simulink model "ban5"  (R2018b)
settings: Solver=FixedStepAuto  StartTime=0.0  StopTime=10  FixedStep=0.001  RelTol=1e-3
libraries: simulink x1
settings Model: Creator=User  LastModifiedBy=User

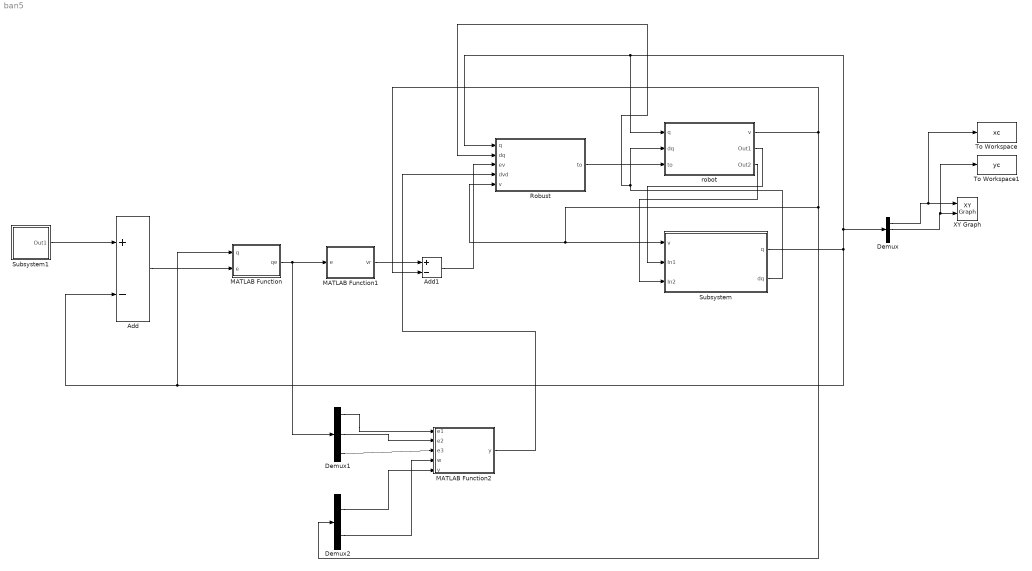
== system ban5 ==
  Add : Sum  Inputs=+-
  Add1 : Sum  Inputs=+-
  Demux : Demux  Outputs=3
  Demux1 : Demux  Outputs=3
  Demux2 : Demux  Outputs=2
  MATLAB Function : MATLAB Function  TreatAsAtomicUnit=on
  MATLAB Function1 : MATLAB Function  TreatAsAtomicUnit=on
  MATLAB Function2 : MATLAB Function  TreatAsAtomicUnit=on
  Robust : Subsystem
  Subsystem : Subsystem
  Subsystem1 : Subsystem
  To Workspace : ToWorkspace  VariableName=xc  SampleTime=-1
  To Workspace1 : ToWorkspace  VariableName=yc  SampleTime=-1
  XY Graph : simulink/Sinks/XY Graph  xmin=-4  xmax=4  ymin=-4  ymax=4  st=0.005
  robot : Subsystem
  wires:
  Subsystem1/1(Out1) -> Add/1
  Subsystem/1(q) -> robot/1(q), Robust/1(q), Demux/1, MATLAB Function/1(q), Add/2
  Add/1 -> MATLAB Function/2(e)
  MATLAB Function/1(qe) -> Demux1/1, MATLAB Function1/1(e)
  robot/1(v) -> Demux2/1, Subsystem/1(v), Robust/5(v), Add1/2
  Add1/1 -> Robust/3(ev)
  Subsystem/2(dq) -> robot/2(dq), Robust/2(dq)
  Demux/1 -> To Workspace/1, XY Graph/1
  Demux/2 -> To Workspace1/1, XY Graph/2
  robot/2(Out1) -> Subsystem/2(In1)
  robot/3(Out2) -> Subsystem/3(In2)
  Demux1/1 -> MATLAB Function2/1(e1)
  Demux1/2 -> MATLAB Function2/2(e2)
  Demux1/3 -> MATLAB Function2/3(e3)
  Demux2/1 -> MATLAB Function2/5(v)
  Demux2/2 -> MATLAB Function2/4(w)
  Robust/1(to) -> robot/3(to)
  MATLAB Function2/1(y) -> Robust/4(dvd)
  MATLAB Function1/1(vr) -> Add1/1

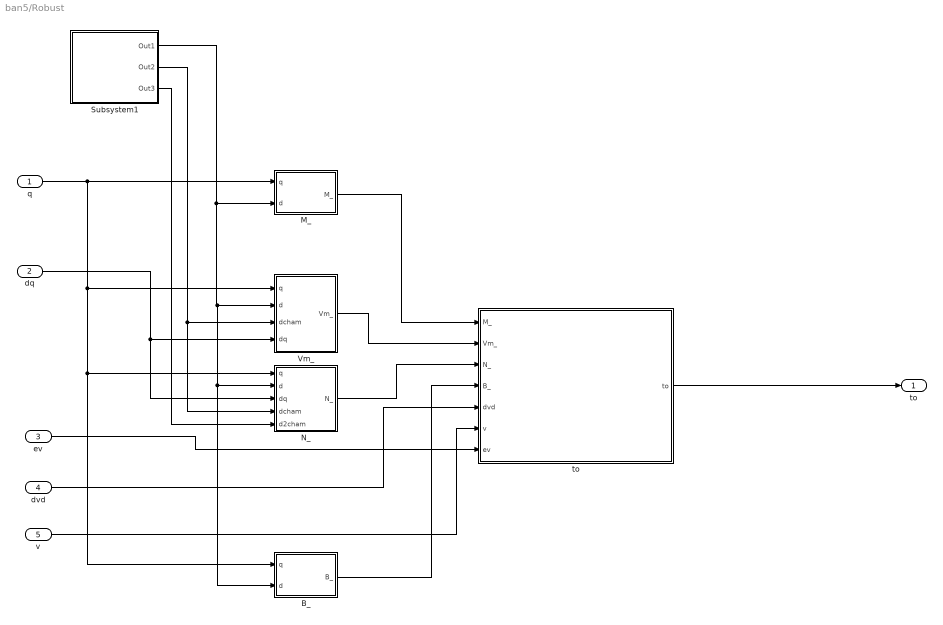
== system ban5/Robust ==
  q : Inport
  dq : Inport  Port=2
  ev : Inport  Port=3
  dvd : Inport  Port=4
  v : Inport  Port=5
  B_ : MATLAB Function  TreatAsAtomicUnit=on
  M_ : MATLAB Function  TreatAsAtomicUnit=on
  N_ : MATLAB Function  TreatAsAtomicUnit=on
  Subsystem1 : Subsystem
  Vm_ : MATLAB Function  TreatAsAtomicUnit=on
  "to " : MATLAB Function  TreatAsAtomicUnit=on
  to : Outport
  wires:
  dq/1 -> Vm_/4(dq), N_/3(dq)
  q/1 -> M_/1(q), Vm_/1(q), N_/1(q), B_/1(q)
  B_/1(B_) -> "to "/4(B_)
  N_/1(N_) -> "to "/3(N_)
  Vm_/1(Vm_) -> "to "/2(Vm_)
  M_/1(M_) -> "to "/1(M_)
  dvd/1 -> "to "/5(dvd)
  v/1 -> "to "/6(v)
  ev/1 -> "to "/7(ev)
  "to "/1(to) -> to/1
  Subsystem1/1(Out1) -> B_/2(d), N_/2(d), Vm_/2(d), M_/2(d)
  Subsystem1/2(Out2) -> N_/4(dcham), Vm_/3(dcham)
  Subsystem1/3(Out3) -> N_/5(d2cham)

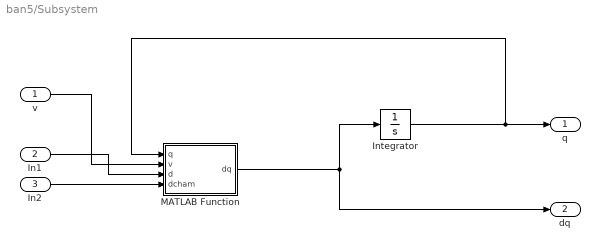
== system ban5/Subsystem ==
  v : Inport
  In1 : Inport  Port=2
  In2 : Inport  Port=3
  Integrator : Integrator  InitialCondition=[1.8852;-0.2772;3*pi/8]
  MATLAB Function : MATLAB Function  TreatAsAtomicUnit=on
  q : Outport
  dq : Outport  Port=2
  wires:
  Integrator/1 -> MATLAB Function/1(q), q/1
  MATLAB Function/1(dq) -> Integrator/1, dq/1
  v/1 -> MATLAB Function/2(v)
  In1/1 -> MATLAB Function/3(d)
  In2/1 -> MATLAB Function/4(dcham)

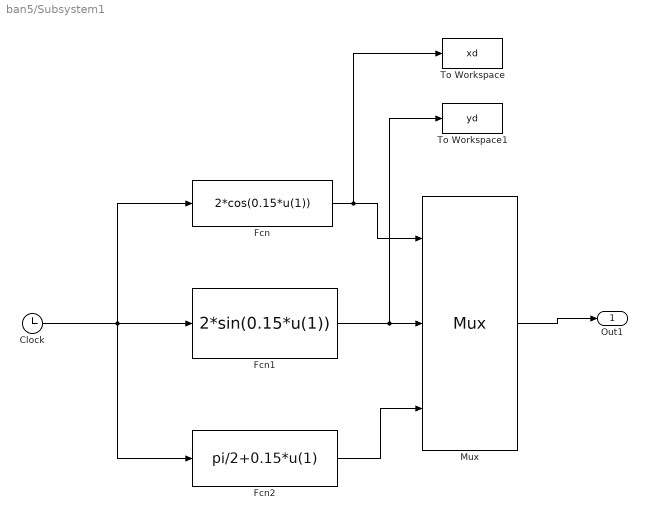
== system ban5/Subsystem1 ==
  Clock : Clock
  Fcn : Fcn  Expr=2*cos(0.15*u(1))
  Fcn1 : Fcn  Expr=2*sin(0.15*u(1))
  Fcn2 : Fcn  Expr=pi/2+0.15*u(1)
  Mux : Mux  Inputs=3
  To Workspace : ToWorkspace  VariableName=xd  SampleTime=-1
  To Workspace1 : ToWorkspace  VariableName=yd  SampleTime=-1
  Out1 : Outport
  wires:
  Clock/1 -> Fcn2/1, Fcn1/1, Fcn/1
  Fcn/1 -> To Workspace/1, Mux/1
  Fcn1/1 -> To Workspace1/1, Mux/2
  Fcn2/1 -> Mux/3
  Mux/1 -> Out1/1

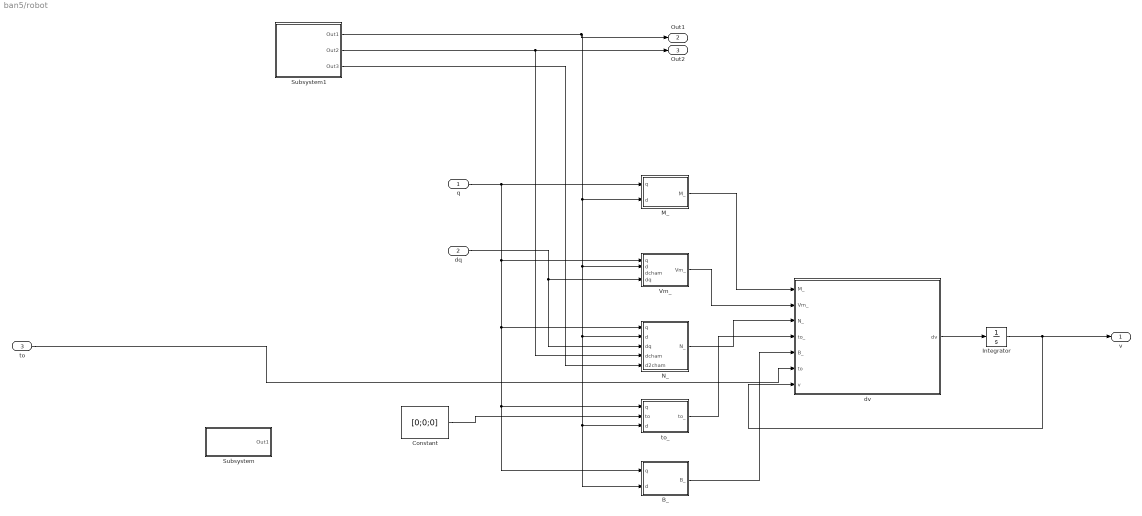
== system ban5/robot ==
  q : Inport
  dq : Inport  Port=2
  to : Inport  Port=3
  B_ : MATLAB Function  TreatAsAtomicUnit=on
  Constant : Constant  Value=[0;0;0]
  Integrator : Integrator  InitialCondition=[0;0]
  M_ : MATLAB Function  TreatAsAtomicUnit=on
  N_ : MATLAB Function  TreatAsAtomicUnit=on
  Subsystem : Subsystem
  Subsystem1 : Subsystem
  Vm_ : MATLAB Function  TreatAsAtomicUnit=on
  dv : MATLAB Function  TreatAsAtomicUnit=on
  to_ : MATLAB Function  TreatAsAtomicUnit=on
  v : Outport
  Out1 : Outport  Port=2
  Out2 : Outport  Port=3
  wires:
  M_/1(M_) -> dv/1(M_)
  Vm_/1(Vm_) -> dv/2(Vm_)
  N_/1(N_) -> dv/3(N_)
  to_/1(to_) -> dv/4(to_)
  B_/1(B_) -> dv/5(B_)
  dv/1(dv) -> Integrator/1
  Integrator/1 -> v/1, dv/7(v)
  q/1 -> B_/1(q), to_/1(q), N_/1(q), Vm_/1(q), M_/1(q)
  dq/1 -> N_/3(dq), Vm_/4(dq)
  to/1 -> dv/6(to)
  Subsystem1/1(Out1) -> Out1/1, B_/2(d), to_/3(d), N_/2(d), Vm_/2(d), M_/2(d)
  Subsystem1/3(Out3) -> N_/5(d2cham)
  Subsystem1/2(Out2) -> Out2/1, N_/4(dcham)
  Constant/1 -> to_/2(to)

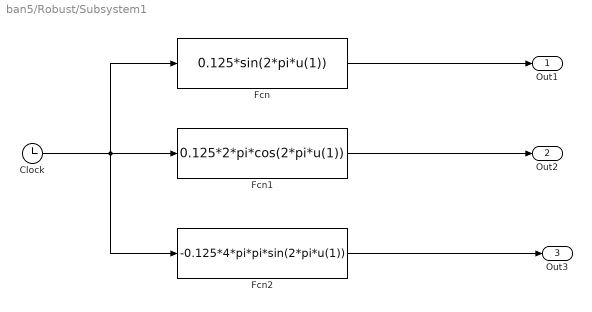
== system ban5/Robust/Subsystem1 ==
  Clock : Clock
  Fcn : Fcn  Expr=0.125*sin(2*pi*u(1))
  Fcn1 : Fcn  Expr=0.125*2*pi*cos(2*pi*u(1))
  Fcn2 : Fcn  Expr=-0.125*4*pi*pi*sin(2*pi*u(1))
  Out1 : Outport
  Out2 : Outport  Port=2
  Out3 : Outport  Port=3
  wires:
  Fcn2/1 -> Out3/1
  Fcn1/1 -> Out2/1
  Fcn/1 -> Out1/1
  Clock/1 -> Fcn2/1, Fcn1/1, Fcn/1

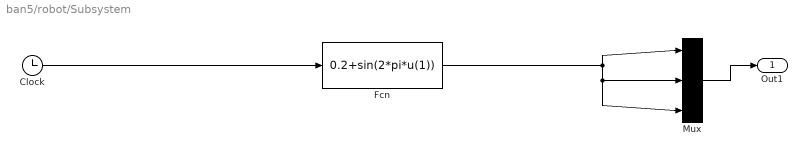
== system ban5/robot/Subsystem ==
  Clock : Clock
  Fcn : Fcn  Expr=0.2+sin(2*pi*u(1))
  Mux : Mux  Inputs=3
  Out1 : Outport
  wires:
  Clock/1 -> Fcn/1
  Fcn/1 -> Mux/3, Mux/2, Mux/1
  Mux/1 -> Out1/1

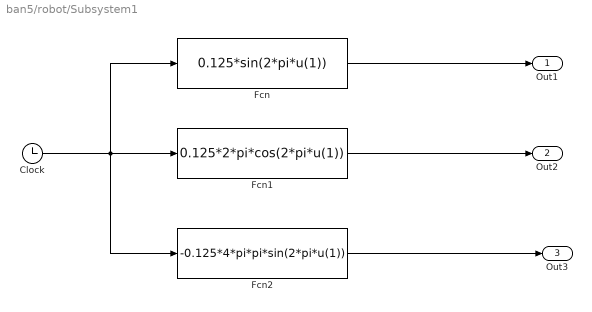
== system ban5/robot/Subsystem1 ==
  Clock : Clock
  Fcn : Fcn  Expr=0.125*sin(2*pi*u(1))
  Fcn1 : Fcn  Expr=0.125*2*pi*cos(2*pi*u(1))
  Fcn2 : Fcn  Expr=-0.125*4*pi*pi*sin(2*pi*u(1))
  Out1 : Outport
  Out2 : Outport  Port=2
  Out3 : Outport  Port=3
  wires:
  Fcn2/1 -> Out3/1
  Fcn1/1 -> Out2/1
  Fcn/1 -> Out1/1
  Clock/1 -> Fcn2/1, Fcn1/1, Fcn/1

== matlab function ban5/MATLAB Function ==
  data: q input; qe output; e input
function qe = fcn(q,e)
phi=q(3);
qe=[cos(phi) sin(phi) 0;-sin(phi) cos(phi) 0;0 0 1]*e;
end

== matlab function ban5/Subsystem/MATLAB Function ==
  data: q input; dq output; v input; d input; dcham input
function dq = fcn(q,v,d,dcham)
phi=[0 0 1]*q;
S=[cos(phi) -d*sin(phi);sin(phi) d*cos(phi);0 1];
n=[dcham*cos(phi);dcham*sin(phi);0];
dq=S*v+n;
end

== matlab function ban5/MATLAB Function1 ==
  data: e input; vr output
function vr=fcn(e)
vr=[0.3*cos([0 0 1]*e)+10*[1 0 0]*e;
    0.15+10*0.3*[0 1 0]*e+10*0.3*sin([0 0 1]*e)];
end

== matlab function ban5/robot/M_ ==
  data: q input; M_ output; d input
function M_ = fcn(q,d)
m=8;
I=0.7075+5*d^2;
M=[m 0 m*d*sin(q(3));
    0 m -m*d*cos(q(3));
    m*d*sin(q(3)) -m*d*cos(q(3)) I];
S=[cos(q(3)) -d*sin(q(3));
    sin(q(3)) d*cos(q(3));
    0 1];
M_=S'*M*S;
end

== matlab function ban5/robot/Vm_ ==
  data: q input; Vm_ output; d input; dcham input; dq input
function Vm_ = fcn(q,d,dcham,dq)
m=8;
I=0.7075+5*d^2;
M=[m 0 m*d*sin(q(3));
    0 m -m*d*cos(q(3));
    m*d*sin(q(3)) -m*d*cos(q(3)) I];
S=[cos(q(3)) -d*sin(q(3));
    sin(q(3)) d*cos(q(3));
    0 1];
dS=[-sin(q(3))*dq(3) -dcham*sin(q(3))-d*cos(q(3))*dq(3);
    cos(q(3))*dq(3) dcham*cos(q(3))-d*sin(q(3))*dq(3);
    0 0];
Vm=[0 0 m*d*dq(3)*cos(q(3));
    0 0 m*d*dq(3)*sin(q(3));
    0 0 0];
Vm_=S'*(M*dS+Vm*S);
end

== matlab function ban5/robot/N_ ==
  data: q input; N_ output; d input; dq input; dcham input; d2cham input
function N_ = fcn(q,d,dq,dcham,d2cham)
m=8;
I=0.7075+5*d^2;
M=[m 0 m*d*sin(q(3));
    0 m -m*d*cos(q(3));
    m*d*sin(q(3)) -m*d*cos(q(3)) I];
S=[cos(q(3)) -d*sin(q(3));
    sin(q(3)) d*cos(q(3));
    0 1];
Vm=[0 0 m*d*dq(3)*cos(q(3));
    0 0 m*d*dq(3)*sin(q(3));
    0 0 0];
n=[dcham*cos(q(3));dcham*sin(q(3));0];
dn=[d2cham*cos(q(3))+dcham*dq(3)*-sin(q(3));
    d2cham*sin(q(3))+dcham*dq(3)*cos(q(3));
    0];
N_=S'*(M*dn+Vm*n);
end

== matlab function ban5/robot/to_ ==
  data: q input; to_ output; to input; d input
function to_ = fcn(q,to,d)
S=[cos(q(3)) -d*sin(q(3));
    sin(q(3)) d*cos(q(3));
    0 1];
to_=S'*to;
end

== matlab function ban5/robot/B_ ==
  data: q input; B_ output; d input
function B_ = fcn(q,d)
S=[cos(q(3)) -d*sin(q(3));
    sin(q(3)) d*cos(q(3));
    0 1];
B=1/0.2*[cos(q(3)) cos(q(3));
    sin(q(3)) sin(q(3));
    0.25 -0.25];
B_=S'*B;
end

== matlab function ban5/robot/dv ==
  data: M_ input; dv output; Vm_ input; N_ input; to_ input; B_ input; to input; v input
function dv = fcn(M_,Vm_,N_,to_,B_,to,v)
dv=M_\(B_*to-to_-N_-Vm_*v);
end

== matlab function ban5/MATLAB Function2 ==
  data: e1 input; y output; e2 input; e3 input; w input; v input
function y = fcn(e1,e2,e3,w,v)
dvd=-0.3*sin(e3)*(0.15-w)+10*(0.3*cos(e3)+w*e2-v);
dwd=10*0.3*(0.3*sin(e3)-w*e1)+10*0.3*(0.15-w)*cos(e3);
y=[dvd;dwd];
end

== matlab function ban5/Robust/B_ ==
  data: q input; B_ output; d input
function B_ = fcn(q,d)
S=[cos(q(3)) -d*sin(q(3));
    sin(q(3)) d*cos(q(3));
    0 1];
B=1/0.2*[cos(q(3)) cos(q(3));
    sin(q(3)) sin(q(3));
    0.25 -0.25];
B_=S'*B;
end

== matlab function ban5/Robust/M_ ==
  data: q input; M_ output; d input
function M_ = fcn(q,d)
m=8;
I=0.7075+5*d^2;
M=[m 0 m*d*sin(q(3));
    0 m -m*d*cos(q(3));
    m*d*sin(q(3)) -m*d*cos(q(3)) I];
S=[cos(q(3)) -d*sin(q(3));
    sin(q(3)) d*cos(q(3));
    0 1];
M_=S'*M*S;
end

== matlab function ban5/Robust/N_ ==
  data: q input; N_ output; d input; dq input; dcham input; d2cham input
function N_ = fcn(q,d,dq,dcham,d2cham)
m=8;
I=0.7075+5*d^2;
M=[m 0 m*d*sin(q(3));
    0 m -m*d*cos(q(3));
    m*d*sin(q(3)) -m*d*cos(q(3)) I];
S=[cos(q(3)) -d*sin(q(3));
    sin(q(3)) d*cos(q(3));
    0 1];
Vm=[0 0 m*d*dq(3)*cos(q(3));
    0 0 m*d*dq(3)*sin(q(3));
    0 0 0];
n=[dcham*cos(q(3));dcham*sin(q(3));0];
dn=[d2cham*cos(q(3))+dcham*dq(3)*-sin(q(3));
    d2cham*sin(q(3))+dcham*dq(3)*cos(q(3));
    0];
N_=S'*(M*dn+Vm*n);
end

== matlab function ban5/Robust/Vm_ ==
  data: q input; Vm_ output; d input; dcham input; dq input
function Vm_ = fcn(q,d,dcham,dq)
m=8;
I=0.7075+5*d^2;
M=[m 0 m*d*sin(q(3));
    0 m -m*d*cos(q(3));
    m*d*sin(q(3)) -m*d*cos(q(3)) I];
S=[cos(q(3)) -d*sin(q(3));
    sin(q(3)) d*cos(q(3));
    0 1];
dS=[-sin(q(3))*dq(3) -dcham*sin(q(3))-d*cos(q(3))*dq(3);
    cos(q(3))*dq(3) dcham*cos(q(3))-d*sin(q(3))*dq(3);
    0 0];
Vm=[0 0 m*d*dq(3)*cos(q(3));
    0 0 m*d*dq(3)*sin(q(3));
    0 0 0];
Vm_=S'*(M*dS+Vm*S);
end

== matlab function ban5/Robust/to  ==
  data: M_ input; to output; Vm_ input; N_ input; B_ input; dvd input; v input; ev input
function to = fcn(M_,Vm_,N_,B_,dvd,v,ev)
s=ev;
sats=[0;0];
if abs(s(1))>0.02
    sats(1)=1;
else
    sats(1)=s(1)*50;
end
if abs(s(2))>0.02
    sats(2)=1;
else
    sats(2)=s(2)*50;
end
to=B_\(M_*dvd+Vm_*v+N_+(20+20)*M_*sats+30*M_*s);
end
